simulink model "doublePendWork2015b"  (Simulink 8.6)
settings: Solver=FixedStepAuto  StartTime=0.0  StopTime=inf  FixedStep=0.002  RelTol=1e-3
values from neighbouring files (symbols this model uses):
  epsilon = deg2rad(20)    [params_calc.m]
  Er = 2*Mp*lp*9.81    (= 1.066090959)    [params_calc.m]
  eta_g = 1    [params_calc.m]
  eta_m = 1    [params_calc.m]
  Euu = f1+f2    [DIP.m]    (also in params_calc.m = 1.066090959)
  g = 9.81    [params_calc.m]
  Jp = Mp * Lp^2 / 12    (= 0.00494556806583)    [params_calc.m]
  K_EC = Pr * N_pp / ( 4 * 1024 )    (= 2.27485440932e-05)    [params_calc.m]
  K_EP = 2 * pi / ( 4 * 1024 )    (= 0.00153398078789)    [params_calc.m]
  Kg = 3.71    [params_calc.m]
  Km = 0.804e-3 * K_RDPS2RPM    (= 0.00767763445475)    [params_calc.m]
  Ks = -1    [DIP.m]
  Kt = 1.088 * K_OZ2N * K_IN2M    (= 0.00768296972928)    [params_calc.m]
  L2 = 0.3365    [params_calc.m]
  lp = Lp/2    (= 0.27305)    [params_calc.m]
  Mc = m0    (= 0.94)    [params_calc.m]
  Mp = m1 + m2    (= 0.199)    [params_calc.m]
  r_mp = 0.5 / 2 * K_IN2M    (= 0.00635)    [params_calc.m]
  Rm = 2.6    [params_calc.m]
  wcf = 2 * pi * 10.0    (= 62.8318530718)    [params_calc.m]
  zetaf = 0.9    [params_calc.m]
undefined symbols (not defined in the file or in its folder): HIL, K
libraries: simulink x5, quarc_library x4, simulink_extras x4
settings Model: Creator=mech2019  LastModifiedBy=User  SimulationMode=external  ExtModeTrigDuration=10000
settings SolverCC: PositivePriorityOrder=on
settings DataIOCC: SaveFormat=Dataset  SignalLoggingSaveFormat=Dataset
settings OptimizationCC: ExpressionDepthLimit=128
settings DebuggingCC: UnderspecifiedInitializationDetection=Simplified  MergeDetectMultiDrivingBlocksExec=error  SolverPrmCheckMsg=none  FcnCallInpInsideContextMsg=EnableAllAsError  StateNameClashWarn=none
settings HardwareCC: ProdBitPerPointer=64  ProdLargestAtomicFloat=Float  ProdIntDivRoundTo=Zero  ProdEndianess=LittleEndian  ProdWordSize=64  ProdHWDeviceType=Intel->x86-64 (Windows64)
settings RTWCC: SystemTargetFile=quarc_win64.tlc  TemplateMakefile=quarc_default_tmf  Description=QUARC Win64 Target
settings STFCustomTargetCC: TargetPreCompLibLocation=C:\PROGRA~3\QUARC\lib\2015b\win64\release  ConcurrentExecutionCompliant=on  SystemTargetFile=quarc_win64.tlc
settings GRTTargetCC: TargetPreCompLibLocation=C:\PROGRA~3\QUARC\lib\2015b\win64\release  ParMdlRefBuildCompliant=off  CompOptLevelCompliant=off  GeneratePreprocessorConditionals=Use local settings  MatFileLogging=off  CPPClassGenCompliant=off  UseToolchainInfoCompliant=off  ExtMode=on  ExtModeMexFile=quarc_comm

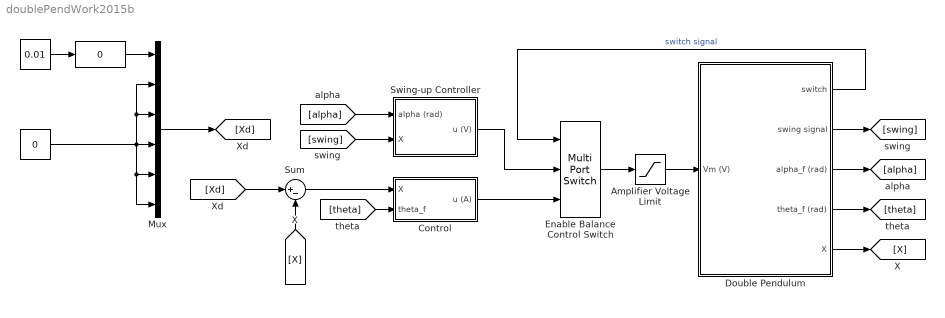
== system doublePendWork2015b ==
  "  " : Constant  Value=0
  "    " : Constant  Value=0.01
  "       " : simulink/Math Operations/Slider Gain  gain=0  low=-200  high=200
  "  Double Pendulum " : Subsystem
      mask Display:
      | image(imread('DIP.jpg'));
      | port_label('input',1,'V');
      | port_label('output',1,'switch');
      | port_label('output',2,'swing');
      | port_label('output',3,'alpha');
      | port_label('output',4,'theta');
      | port_label('output',5,'X');
  Amplifier Voltage Limit : Saturate  UpperLimit=6  LowerLimit=-6
  Control : Subsystem
  Enable Balance Control Switch : MultiPortSwitch  DataPortOrder=Zero-based contiguous  Inputs=2  zeroidx=on
  Mux : Mux  Inputs=6
  Sum : Sum  Inputs=|+-
  Swing-up Controller : Subsystem
  wires:
  Enable Balance Control Switch/1 -> Amplifier Voltage Limit/1
  Amplifier Voltage Limit/1 -> "  Double Pendulum "/1(Vm (V))
  Swing-up Controller/1(u (V)) -> Enable Balance Control Switch/2
  "  Double Pendulum "/1(switch) -> Enable Balance Control Switch/1  "switch signal"
  Control/1(u (A)) -> Enable Balance Control Switch/3
  Sum/1 -> Control/1(X)
  "    "/1 -> "       "/1
  "  "/1 -> Mux/6, Mux/5, Mux/2, Mux/3, Mux/4
  [Xd] -> Sum/1
  "       "/1 -> Mux/1
  Mux/1 -> [Xd]
  "  Double Pendulum "/5(X) -> [X]
  [X] -> Sum/2
  "  Double Pendulum "/4(theta_f (rad)) -> [theta]
  [theta] -> Control/2(theta_f)
  [swing] -> Swing-up Controller/2(X)
  "  Double Pendulum "/2(swing signal) -> [swing]
  "  Double Pendulum "/3(alpha_f (rad)) -> [alpha]
  [alpha] -> Swing-up Controller/1(alpha (rad))

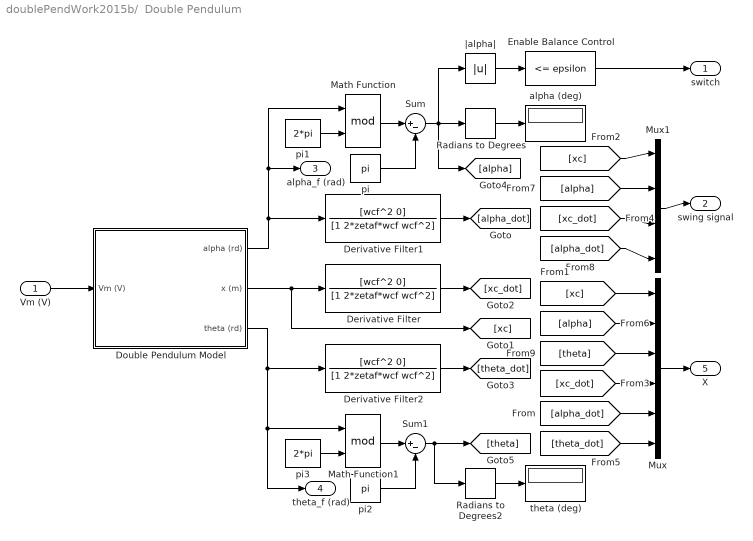
== system doublePendWork2015b/  Double Pendulum  ==
  Vm (V) : Inport
  Derivative Filter : TransferFcn  Numerator=[wcf^2 0]  Denominator=[1 2*zetaf*wcf wcf^2]
  Derivative Filter1 : TransferFcn  Numerator=[wcf^2 0]  Denominator=[1 2*zetaf*wcf wcf^2]
  Derivative Filter2 : TransferFcn  Numerator=[wcf^2 0]  Denominator=[1 2*zetaf*wcf wcf^2]
  Double Pendulum Model : Subsystem
  Enable Balance Control : simulink/Logic and Bit Operations/Compare To Constant  relop=<=  const=epsilon  OutDataTypeStr=uint8  ZeroCross=off
  Math Function : Math  Operator=mod  SaturateOnIntegerOverflow=on
  Math Function1 : Math  Operator=mod  SaturateOnIntegerOverflow=on
  Mux : Mux  Inputs=6
  Mux1 : Mux
  Radians to Degrees : simulink_extras/Transformations/Radians to Degrees
  Radians to Degrees2 : simulink_extras/Transformations/Radians to Degrees
  Sum : Sum  Inputs=|+-  SaturateOnIntegerOverflow=on  InputSameDT=on  OutDataTypeStr=Inherit: Same as first input
  Sum1 : Sum  Inputs=|+-  SaturateOnIntegerOverflow=on  InputSameDT=on  OutDataTypeStr=Inherit: Same as first input
  alpha (deg) : Display
      settings: Decimation=100
  pi : Constant  Value=pi
  pi1 : Constant  Value=2*pi
  pi2 : Constant  Value=pi
  pi3 : Constant  Value=2*pi
  theta (deg) : Display
      settings: Decimation=100
  |alpha| : Abs
  switch : Outport  InitialOutput=0
  swing signal : Outport  Port=2  InitialOutput=0
  alpha_f (rad) : Outport  Port=3  InitialOutput=0
  theta_f (rad) : Outport  Port=4  InitialOutput=0
  X : Outport  Port=5  InitialOutput=0
  wires:
  Double Pendulum Model/2(x (m)) -> [xc], Derivative Filter/1
  Derivative Filter/1 -> [xc_dot]
  pi1/1 -> Math Function/2
  Vm (V)/1 -> Double Pendulum Model/1(Vm (V))
  pi/1 -> Sum/2
  Math Function/1 -> Sum/1
  Derivative Filter2/1 -> [theta_dot]
  pi3/1 -> Math Function1/2
  pi2/1 -> Sum1/2
  Math Function1/1 -> Sum1/1
  Sum1/1 -> [theta], Radians to Degrees2/1
  Double Pendulum Model/1(alpha (rd)) -> Math Function/1, alpha_f (rad)/1, Derivative Filter1/1
  Radians to Degrees2/1 -> theta (deg)/1
  Double Pendulum Model/3("theta (rd) ") -> Derivative Filter2/1, Math Function1/1, theta_f (rad)/1
  Mux/1 -> X/1
  Derivative Filter1/1 -> [alpha_dot]
  Mux1/1 -> swing signal/1
  |alpha|/1 -> Enable Balance Control/1
  Enable Balance Control/1 -> switch/1
  Sum/1 -> |alpha|/1, Radians to Degrees/1, [alpha]
  [alpha_dot] -> Mux/5
  [xc] -> Mux/1
  [xc] -> Mux1/1
  [xc_dot] -> Mux/4
  [xc_dot] -> Mux1/3
  [theta_dot] -> Mux/6
  [alpha] -> Mux/2
  [alpha] -> Mux1/2
  [alpha_dot] -> Mux1/4
  [theta] -> Mux/3
  Radians to Degrees/1 -> alpha (deg)/1

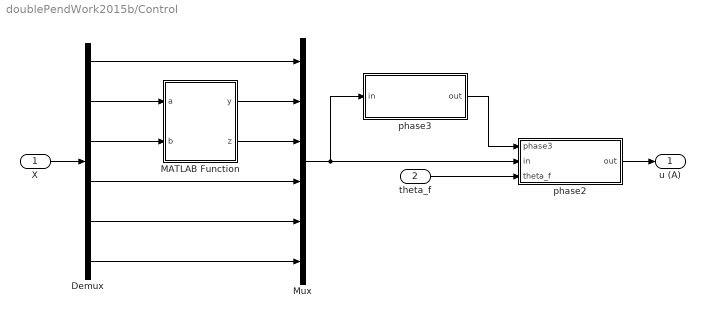
== system doublePendWork2015b/Control ==
  X : Inport
  theta_f : Inport  Port=2
  Demux : Demux  Outputs=6
  MATLAB Function : MATLAB Function  TreatAsAtomicUnit=on
  Mux : Mux  Inputs=6
  phase2 : Subsystem
  phase3 : Subsystem
  u (A) : Outport
  wires:
  X/1 -> Demux/1
  phase2/1(out) -> u (A)/1
  Demux/2 -> MATLAB Function/1(a)
  Demux/3 -> MATLAB Function/2(b)
  MATLAB Function/2(z) -> Mux/3
  MATLAB Function/1(y) -> Mux/2
  Demux/1 -> Mux/1
  Demux/4 -> Mux/4
  Demux/5 -> Mux/5
  Demux/6 -> Mux/6
  Mux/1 -> phase2/2(in), phase3/1(in)
  phase3/1(out) -> phase2/1(phase3)
  theta_f/1 -> phase2/3(theta_f)

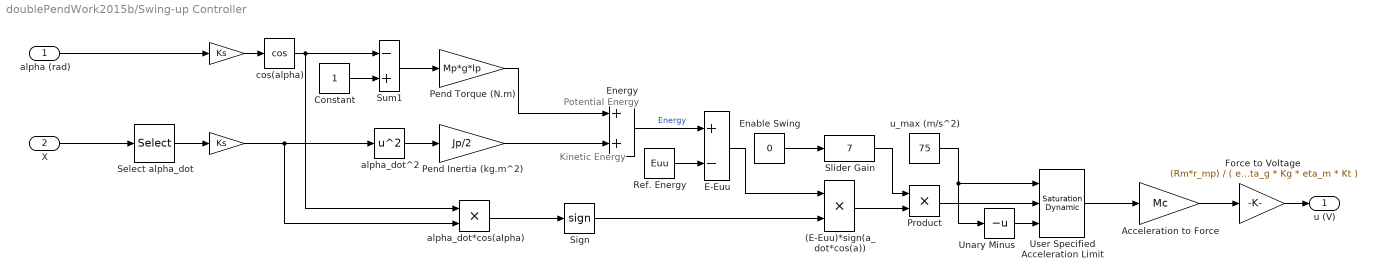
== system doublePendWork2015b/Swing-up Controller ==
  note: Potential Energy
  note: Kinetic Energy
  alpha (rad) : Inport
  X : Inport  Port=2
  "    " : Gain  Gain=Ks
  "           " : Gain  Gain=Ks
  (E-Euu)*sign(a_dot*cos(a)) : Product  RndMeth=Zero
  Acceleration to Force : Gain  Gain=Mc
  Constant : Constant
  E-Euu : Sum  Inputs=+-
  Enable Swing : Constant  Value=0
  Energy : Sum  SaturateOnIntegerOverflow=on
  Force to Voltage : Gain  Gain=(Rm*r_mp) / ( eta_g * Kg * eta_m * Kt )
  Pend Inertia (kg.m^2) : Gain  Gain=Jp/2
  Pend Torque (N.m) : Gain  Gain=Mp*g*lp
  Product : Product  RndMeth=Zero
  Ref. Energy : Constant  Value=Euu
  Select alpha_dot : Selector  InputPortWidth=4  IndexOptions=Index vector (dialog)  Indices=[4]  OutputSizes=1
  Sign : Signum
  Slider Gain : simulink/Math Operations/Slider Gain  gain=7  low=0  high=200
  Sum1 : Sum  Inputs=-+  SaturateOnIntegerOverflow=on
  Unary Minus : UnaryMinus
  User Specified Acceleration Limit : simulink/Discontinuities/Saturation Dynamic  OutMin=[]  OutMax=[]  OutDataTypeStr=Inherit: Same as second input  OutDataType=fixdt(1, 16)  OutScaling=2^-10  DoSatur=off
  alpha_dot*cos(alpha) : Product  RndMeth=Zero
  alpha_dot^2 : Math  Operator=square  SaturateOnIntegerOverflow=on
  cos(alpha) : Trigonometry  Operator=cos
  u_max (m/s^2) : Constant  Value=75
  u (V) : Outport
  wires:
  User Specified Acceleration Limit/1 -> Acceleration to Force/1
  Acceleration to Force/1 -> Force to Voltage/1
  alpha (rad)/1 -> "    "/1
  Select alpha_dot/1 -> "           "/1
  X/1 -> Select alpha_dot/1
  Force to Voltage/1 -> u (V)/1
  Enable Swing/1 -> Slider Gain/1
  Energy/1 -> E-Euu/1  "Energy"
  alpha_dot^2/1 -> Pend Inertia (kg.m^2)/1
  Constant/1 -> Sum1/2
  cos(alpha)/1 -> Sum1/1, alpha_dot*cos(alpha)/1
  Unary Minus/1 -> User Specified Acceleration Limit/3
  Pend Torque (N.m)/1 -> Energy/1
  Ref. Energy/1 -> E-Euu/2
  "           "/1 -> alpha_dot*cos(alpha)/2, alpha_dot^2/1
  E-Euu/1 -> (E-Euu)*sign(a_dot*cos(a))/1
  u_max (m/s^2)/1 -> User Specified Acceleration Limit/1, Unary Minus/1
  (E-Euu)*sign(a_dot*cos(a))/1 -> Product/2
  Sign/1 -> (E-Euu)*sign(a_dot*cos(a))/2
  Product/1 -> User Specified Acceleration Limit/2
  "    "/1 -> cos(alpha)/1
  alpha_dot*cos(alpha)/1 -> Sign/1
  Pend Inertia (kg.m^2)/1 -> Energy/2
  Sum1/1 -> Pend Torque (N.m)/1
  Slider Gain/1 -> Product/1

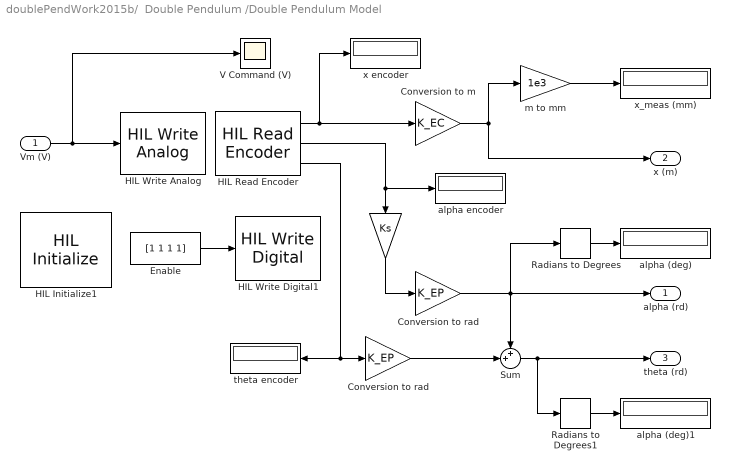
== system doublePendWork2015b/  Double Pendulum /Double Pendulum Model ==
  Vm (V) : Inport
  "    " : Gain  Gain=Ks
  Conversion to m : Gain  Gain=K_EC  SaturateOnIntegerOverflow=on  OutDataTypeStr=Inherit: Same as input  ParamDataTypeStr=Inherit: Same as input
  Conversion to rad : Gain  Gain=K_EP  SaturateOnIntegerOverflow=on  OutDataTypeStr=Inherit: Same as input  ParamDataTypeStr=Inherit: Same as input
  "Conversion to rad " : Gain  Gain=K_EP  SaturateOnIntegerOverflow=on  OutDataTypeStr=Inherit: Same as input  ParamDataTypeStr=Inherit: Same as input
  "Enable " : Constant  Value=[1 1 1 1]
  HIL Initialize1 : quarc_library/Data Acquisition/Generic/Configuration/HIL Initialize  Priority=-99  object_name=HIL-2  board_type=q4  board_number=0  board_options=""  exclusive=off  active=off  hardware_clocks=[0:1]  clock_modes=[0 0]  initial_clock_frequencies=[]  set_clock_params_at_start=on  set_clock_params_at_switch_in=off  set_clock_frequencies_at_start=off  set_clock_frequencies_at_switch_in=off  analog_input_channels=[0:3]  analog_input_maximums=10  analog_input_minimums=-10  set_analog_input_params_at_start=off  set_analog_input_params_at_switch_in=off  analog_output_channels=[0:3]  analog_output_maximums=[10]  analog_output_minimums=[-10]  initial_analog_outputs=[0]  final_analog_outputs=[0]  watchdog_analog_outputs=0  set_analog_output_params_at_start=on  set_analog_output_params_at_switch_in=off  set_analog_outputs_at_start=on  set_analog_outputs_at_switch_in=off  set_analog_outputs_at_terminate=on  set_analog_outputs_at_switch_out=off  set_analog_outputs_on_watchdog=off  digital_input_channels=[]  digital_output_channels=[]  digital_output_configuration=[]  initial_digital_outputs=[1]  final_digital_outputs=[1]  watchdog_digital_outputs=[2]  set_digital_output_params_at_start=off  set_digital_output_params_at_switch_in=off  set_digital_outputs_at_start=on  set_digital_outputs_at_switch_in=off  set_digital_outputs_at_terminate=on  set_digital_outputs_at_switch_out=off  set_digital_outputs_on_watchdog=off  encoder_channels=[0:3]  quadrature=[4]  encoder_filter_frequency=(1/60e-9)/1  initial_encoder_counts=[0]  set_encoder_params_at_start=on  set_encoder_params_at_switch_in=off  set_encoder_counts_at_start=on  set_encoder_counts_at_switch_in=off  pwm_channels=[]  pwm_modes=[0]  pwm_frequency=(1/60e-9)/1024  pwm_configuration=[]  pwm_alignment=[]  pwm_polarity=[]  pwm_leading_deadband=[]  pwm_trailing_deadband=[]  initial_pwm_outputs=[0]  final_pwm_outputs=[0]  watchdog_pwm_outputs=[]  set_pwm_params_at_start=on  set_pwm_params_at_switch_in=off  set_pwm_outputs_at_start=on  set_pwm_outputs_at_switch_in=off  set_pwm_outputs_at_terminate=on  set_pwm_outputs_at_switch_out=off  set_pwm_outputs_on_watchdog=off  other_output_channels=[]  initial_other_outputs=[]  final_other_outputs=[]  watchdog_other_outputs=[]  set_other_outputs_at_start=off  set_other_outputs_at_switch_in=off  set_other_outputs_at_terminate=off  set_other_outputs_at_switch_out=off  set_other_outputs_on_watchdog=off
  HIL Read Encoder : quarc_library/Data Acquisition/Generic/Immediate I//O/HIL Read Encoder  object_name=HIL-2  channels=[3 1 2]  sample_time=qc_get_step_size  active=on  vector_output=off  data_type_mode=Inherit via back propagation  data_type=double
  HIL Write Analog : quarc_library/Data Acquisition/Generic/Immediate I//O/HIL Write Analog  object_name=HIL-2  channels=0  sample_time=-1  active=off  vector_input=off
  HIL Write Digital1 : quarc_library/Data Acquisition/Generic/Immediate I//O/HIL Write Digital  object_name=HIL-2  channels=[0:3]  sample_time=-1  active=off  vector_input=on
  Radians to Degrees : simulink_extras/Transformations/Radians to Degrees
  Radians to Degrees1 : simulink_extras/Transformations/Radians to Degrees
  Sum : Sum  Inputs=++|
  V Command (V) : Scope
  alpha (deg) : Display
      settings: Decimation=100
  alpha (deg)1 : Display
      settings: Decimation=100
  alpha encoder : Display
      settings: Decimation=100
  m to mm : Gain  Gain=1e3  SaturateOnIntegerOverflow=on  OutDataTypeStr=Inherit: Same as input  ParamDataTypeStr=Inherit: Same as input
  "theta encoder " : Display
      settings: Decimation=100
  x encoder : Display
      settings: Decimation=100
  x_meas (mm) : Display
      settings: Decimation=100
  alpha (rd) : Outport  InitialOutput=0
  x (m) : Outport  Port=2  InitialOutput=0
  "theta (rd) " : Outport  Port=3  InitialOutput=0
  wires:
  HIL Read Encoder/1 -> x encoder/1, Conversion to m/1
  Conversion to m/1 -> x (m)/1, m to mm/1
  m to mm/1 -> x_meas (mm)/1
  HIL Read Encoder/2 -> "    "/1, alpha encoder/1
  Radians to Degrees/1 -> alpha (deg)/1
  Vm (V)/1 -> V Command (V)/1, HIL Write Analog/1
  "Enable "/1 -> HIL Write Digital1/1
  "Conversion to rad "/1 -> Sum/2
  "    "/1 -> Conversion to rad/1
  HIL Read Encoder/3 -> "Conversion to rad "/1, "theta encoder "/1
  Radians to Degrees1/1 -> alpha (deg)1/1
  Sum/1 -> "theta (rd) "/1, Radians to Degrees1/1
  Conversion to rad/1 -> alpha (rd)/1, Radians to Degrees/1, Sum/1

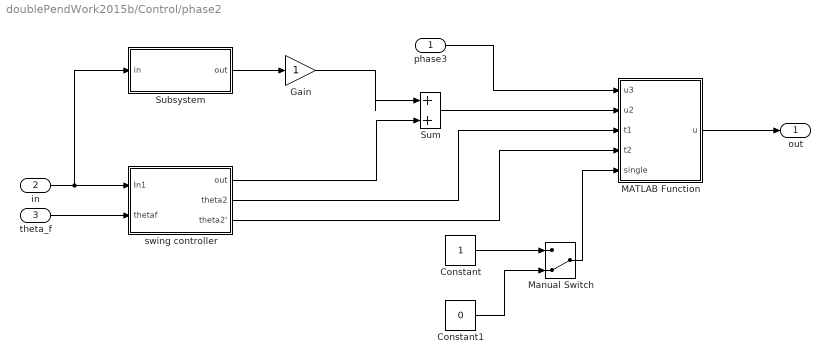
== system doublePendWork2015b/Control/phase2 ==
  phase3 : Inport
  in : Inport  Port=2
  theta_f : Inport  Port=3
  Constant : Constant
  Constant1 : Constant  Value=0
  Gain : Gain
  MATLAB Function : MATLAB Function  TreatAsAtomicUnit=on
  Manual Switch : ManualSwitch  CurrentSetting=0
  Subsystem : Subsystem
  Sum : Sum  Inputs=|++
  swing controller : Subsystem
  out : Outport
  wires:
  in/1 -> swing controller/1(In1), Subsystem/1(in)
  Subsystem/1(out) -> Gain/1
  Gain/1 -> Sum/1
  swing controller/1(out) -> Sum/2
  swing controller/2(theta2) -> MATLAB Function/3(t1)
  MATLAB Function/1(u) -> out/1
  Sum/1 -> MATLAB Function/2(u2)
  phase3/1 -> MATLAB Function/1(u3)
  swing controller/3(theta2') -> MATLAB Function/4(t2)
  theta_f/1 -> swing controller/2(thetaf)
  Manual Switch/1 -> MATLAB Function/5(single)
  Constant/1 -> Manual Switch/1
  Constant1/1 -> Manual Switch/2

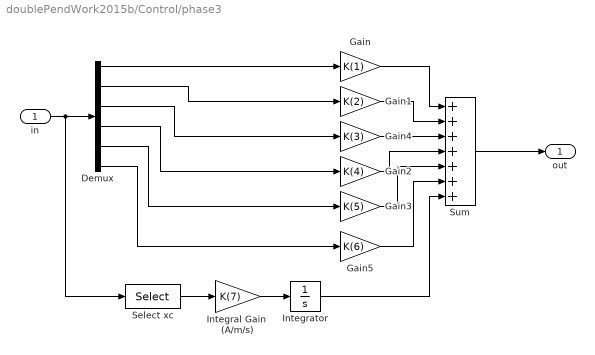
== system doublePendWork2015b/Control/phase3 ==
  in : Inport
  Demux : Demux  Outputs=6
  Gain : Gain  Gain=K(1)
  Gain1 : Gain  Gain=K(2)
  Gain2 : Gain  Gain=K(4)
  Gain3 : Gain  Gain=K(5)
  Gain4 : Gain  Gain=K(3)
  Gain5 : Gain  Gain=K(6)
  Integral Gain  (A/m/s) : Gain  Gain=K(7)
  Integrator : Integrator
  Select xc : Selector  InputPortWidth=6  IndexOptions=Index vector (dialog)  Indices=1  OutputSizes=1
  Sum : Sum  Inputs=+++++++
  out : Outport
  wires:
  Sum/1 -> out/1
  Demux/4 -> Gain2/1
  Demux/2 -> Gain1/1
  Demux/1 -> Gain/1
  Demux/5 -> Gain3/1
  in/1 -> Select xc/1, Demux/1
  Demux/3 -> Gain4/1
  Demux/6 -> Gain5/1
  Gain5/1 -> Sum/6
  Gain3/1 -> Sum/5
  Gain2/1 -> Sum/4
  Gain4/1 -> Sum/3
  Gain1/1 -> Sum/2
  Gain/1 -> Sum/1
  Select xc/1 -> Integral Gain  (A/m/s)/1
  Integral Gain  (A/m/s)/1 -> Integrator/1
  Integrator/1 -> Sum/7

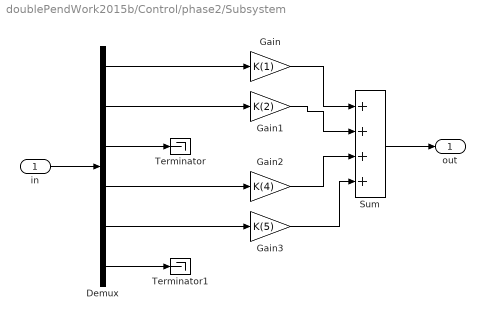
== system doublePendWork2015b/Control/phase2/Subsystem ==
  in : Inport
  Demux : Demux  Outputs=6
  Gain : Gain  Gain=K(1)
  Gain1 : Gain  Gain=K(2)
  Gain2 : Gain  Gain=K(4)
  Gain3 : Gain  Gain=K(5)
  Sum : Sum  Inputs=++++
  Terminator : Terminator
  Terminator1 : Terminator
  out : Outport
  wires:
  in/1 -> Demux/1
  Demux/1 -> Gain/1
  Demux/2 -> Gain1/1
  Demux/5 -> Gain3/1
  Demux/4 -> Gain2/1
  Sum/1 -> out/1
  Gain2/1 -> Sum/3
  Gain3/1 -> Sum/4
  Gain1/1 -> Sum/2
  Gain/1 -> Sum/1
  Demux/3 -> Terminator/1
  Demux/6 -> Terminator1/1

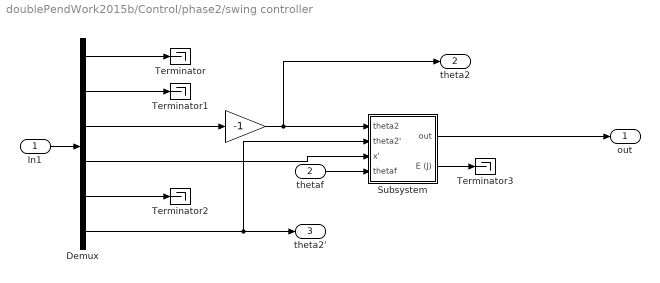
== system doublePendWork2015b/Control/phase2/swing controller ==
  In1 : Inport
  thetaf : Inport  Port=2
  "   " : Gain  Gain=-1
  Demux : Demux  Outputs=6
  Subsystem : Subsystem
  Terminator{,1..3} (4 alike) : Terminator
  out : Outport
  theta2 : Outport  Port=2
  theta2' : Outport  Port=3
  wires:
  In1/1 -> Demux/1
  Demux/3 -> "   "/1
  Demux/6 -> Subsystem/2(theta2'), theta2'/1
  Subsystem/1("out ") -> out/1
  Demux/1 -> Terminator/1
  Demux/4 -> Subsystem/3(x')
  Demux/2 -> Terminator1/1
  Demux/5 -> Terminator2/1
  Subsystem/2(E (J)) -> Terminator3/1
  thetaf/1 -> Subsystem/4(thetaf)
  "   "/1 -> theta2/1, Subsystem/1(theta2)

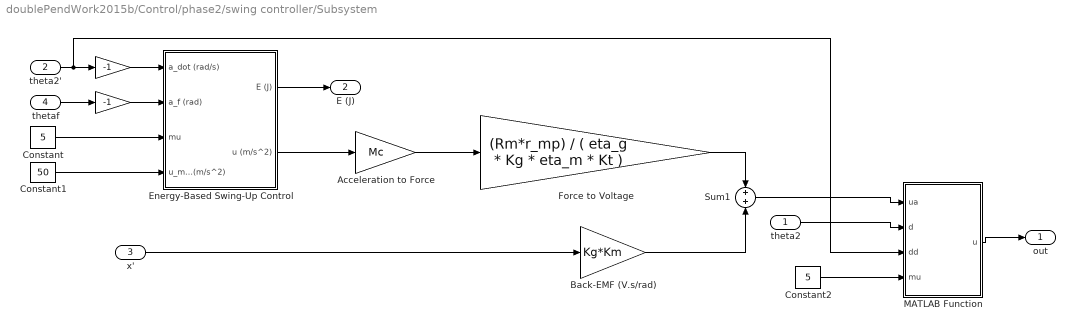
== system doublePendWork2015b/Control/phase2/swing controller/Subsystem ==
  theta2 : Inport
  theta2' : Inport  Port=2
  x' : Inport  Port=3
  thetaf : Inport  Port=4
  "    " : Gain  Gain=-1
  "           " : Gain  Gain=-1
  Acceleration to Force : Gain  Gain=Mc
  Back-EMF (V.s/rad) : Gain  Gain=Kg*Km
  Constant : Constant  Value=5
  Constant1 : Constant  Value=50
  Constant2 : Constant  Value=5
  Energy-Based Swing-Up Control : Subsystem
  Force to Voltage : Gain  Gain=(Rm*r_mp) / ( eta_g * Kg * eta_m * Kt )
  MATLAB Function : MATLAB Function  TreatAsAtomicUnit=on
  Sum1 : Sum
  "out " : Outport
  E (J) : Outport  Port=2
  wires:
  Sum1/1 -> MATLAB Function/1(ua)
  Constant/1 -> Energy-Based Swing-Up Control/3(mu)
  MATLAB Function/1(u) -> "out "/1
  Energy-Based Swing-Up Control/2(u (m/s^2)) -> Acceleration to Force/1
  Acceleration to Force/1 -> Force to Voltage/1
  Energy-Based Swing-Up Control/1(E (J)) -> E (J)/1
  theta2'/1 -> MATLAB Function/3(dd), "           "/1
  Constant1/1 -> Energy-Based Swing-Up Control/4(u_max (m/s^2))
  x'/1 -> Back-EMF (V.s/rad)/1
  Force to Voltage/1 -> Sum1/1
  Back-EMF (V.s/rad)/1 -> Sum1/2
  "    "/1 -> Energy-Based Swing-Up Control/2(a_f (rad))
  "           "/1 -> Energy-Based Swing-Up Control/1(a_dot (rad/s))
  thetaf/1 -> "    "/1
  theta2/1 -> MATLAB Function/2(d)
  Constant2/1 -> MATLAB Function/4(mu)

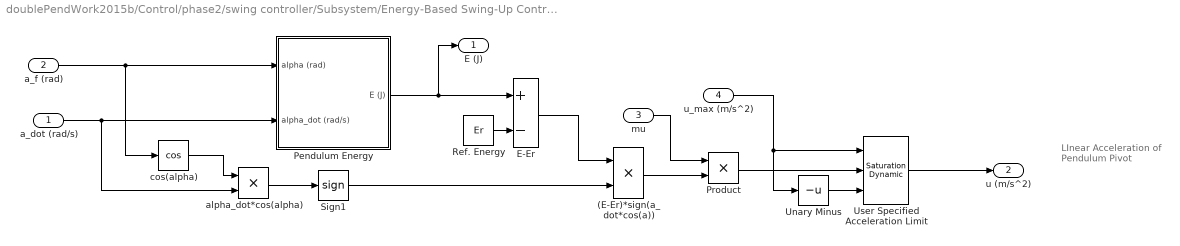
== system doublePendWork2015b/Control/phase2/swing controller/Subsystem/Energy-Based Swing-Up Control ==
  note: LInear Acceleration of
      | Pendulum Pivot
  a_dot (rad/s) : Inport
  a_f (rad) : Inport  Port=2
  mu : Inport  Port=3
  u_max (m/s^2) : Inport  Port=4
  (E-Er)*sign(a_dot*cos(a)) : Product  RndMeth=Zero
  E-Er : Sum  Inputs=+-
  Pendulum Energy : Subsystem
  Product : Product  RndMeth=Zero
  Ref. Energy : Constant  Value=Er
  Sign1 : Signum
  Unary Minus : UnaryMinus
  User Specified Acceleration Limit : simulink/Discontinuities/Saturation Dynamic  OutMin=[]  OutMax=[]  OutDataTypeStr=Inherit: Same as second input  OutDataType=fixdt(1, 16)  OutScaling=2^-10  DoSatur=off
  alpha_dot*cos(alpha) : Product  RndMeth=Zero
  cos(alpha) : Trigonometry  Operator=cos
  E (J) : Outport
  u (m/s^2) : Outport  Port=2
  wires:
  a_f (rad)/1 -> Pendulum Energy/1(alpha (rad)), cos(alpha)/1
  E-Er/1 -> (E-Er)*sign(a_dot*cos(a))/1
  Pendulum Energy/1(E (J)) -> E (J)/1, E-Er/1
  (E-Er)*sign(a_dot*cos(a))/1 -> Product/2
  Ref. Energy/1 -> E-Er/2
  mu/1 -> Product/1
  Product/1 -> User Specified Acceleration Limit/2
  u_max (m/s^2)/1 -> User Specified Acceleration Limit/1, Unary Minus/1
  Unary Minus/1 -> User Specified Acceleration Limit/3
  User Specified Acceleration Limit/1 -> u (m/s^2)/1
  alpha_dot*cos(alpha)/1 -> Sign1/1
  Sign1/1 -> (E-Er)*sign(a_dot*cos(a))/2
  cos(alpha)/1 -> alpha_dot*cos(alpha)/1
  a_dot (rad/s)/1 -> Pendulum Energy/2(alpha_dot (rad/s)), alpha_dot*cos(alpha)/2

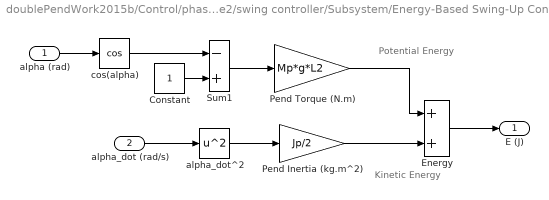
== system doublePendWork2015b/Control/phase2/swing controller/Subsystem/Energy-Based Swing-Up Control/Pendulum Energy ==
  note: Kinetic Energy
  note: Potential Energy
  alpha (rad) : Inport
  alpha_dot (rad/s) : Inport  Port=2
  Constant : Constant
  Energy : Sum  SaturateOnIntegerOverflow=on
  Pend Inertia (kg.m^2) : Gain  Gain=Jp/2
  Pend Torque (N.m) : Gain  Gain=Mp*g*L2
  Sum1 : Sum  Inputs=-+  SaturateOnIntegerOverflow=on
  alpha_dot^2 : Math  Operator=square  SaturateOnIntegerOverflow=on
  cos(alpha) : Trigonometry  Operator=cos
  E (J) : Outport
  wires:
  Constant/1 -> Sum1/2
  Pend Inertia (kg.m^2)/1 -> Energy/2
  Sum1/1 -> Pend Torque (N.m)/1
  alpha_dot^2/1 -> Pend Inertia (kg.m^2)/1
  Pend Torque (N.m)/1 -> Energy/1
  alpha (rad)/1 -> cos(alpha)/1
  alpha_dot (rad/s)/1 -> alpha_dot^2/1
  Energy/1 -> E (J)/1
  cos(alpha)/1 -> Sum1/1

== matlab function Control/MATLAB Function ==
  data: a input double; y output double; b input double; z output double
function [y,z] = fcn(a,b)



y=a;
z=b;

== matlab function Control/phase2/MATLAB Function ==
  data: u3 input double; u output double; u2 input double; t1 input double; t2 input double; single input double
function u = fcn(u3,u2,t1,t2,single)

if (cos(t1)>0.97)&&(abs(t2)<=5)
    u=u3;
else
    u=u2;
end

if(single)
    u=u3; 
end
% (cos(t1)>0.955)&&(abs(t2)<=0.25)
% cos(t1)>0.97

== matlab function Control/phase2/swing controller/Subsystem/MATLAB Function ==
  data: ua input double; u output double; d input double; dd input double; mu input double
function u = fcn(ua,d,dd,mu)

if ((sin(d)*dd)<0)&&(cos(d)<cos(mu))
    u=ua;
else
    u=0;
end
